simulink model "BESTROBITCS_in_output2"  (R2019b)
settings: Solver=FixedStepAuto  StartTime=0.0  StopTime=inf  RelTol=1e-3
libraries: vexarmcortexlib x32, vexcommonlib x6
settings Model: ExtModeTrigDuration=25  Creator=nicoa  LastModifiedBy=nicoa
settings OptimizationCC: EnhancedBackFolding=on  PassReuseOutputArgsAs=Individual arguments  ZeroExternalMemoryAtStartup=off  ZeroInternalMemoryAtStartup=off  MaxStackSize=64  OptimizeBlockOrder=speed  DifferentSizesBufferReuse=on  OptimizationCustomize=off  EfficientTunableParamExpr=on
settings DebuggingCC: ParameterTunabilityLossMsg=error
settings HardwareCC: ProdBitPerPointer=32  ProdBitPerSizeT=32  ProdBitPerPtrDiffT=32  ProdLargestAtomicInteger=Long  ProdLargestAtomicFloat=Double  ProdWordSize=32  ProdHWDeviceType=ARM Compatible->ARM Cortex
settings SFSimCC: MATLABDynamicMemAlloc=off
settings RTWCC: SystemTargetFile=ert.tlc  HardwareBoard=ARM Cortex-based VEX Microcontroller  TLCOptions="-aInlineSetEventsForThisBaseRateFcn=TLC_FALSE -aSuppressMultiTaskScheduler=TLC_FALSE  -aRateBasedStepFcn=0"  TemplateMakefile=ert_default_tmf  GenerateReport=on  Toolchain=GNU Tools for VEX ARM Cortex  IncludeHyperlinkInReport=on  LaunchReport=on  GenerateTraceInfo=on  GenerateTraceReport=on  GenerateTraceReportSl=on  GenerateTraceReportSf=on  GenerateTraceReportEml=on
settings CodeAppCC: ForceParamTrailComments=on  IgnoreCustomStorageClasses=off  OperatorAnnotations=on  SimulinkDataObjDesc=on  SFDataObjDesc=on  InsertBlockDesc=on

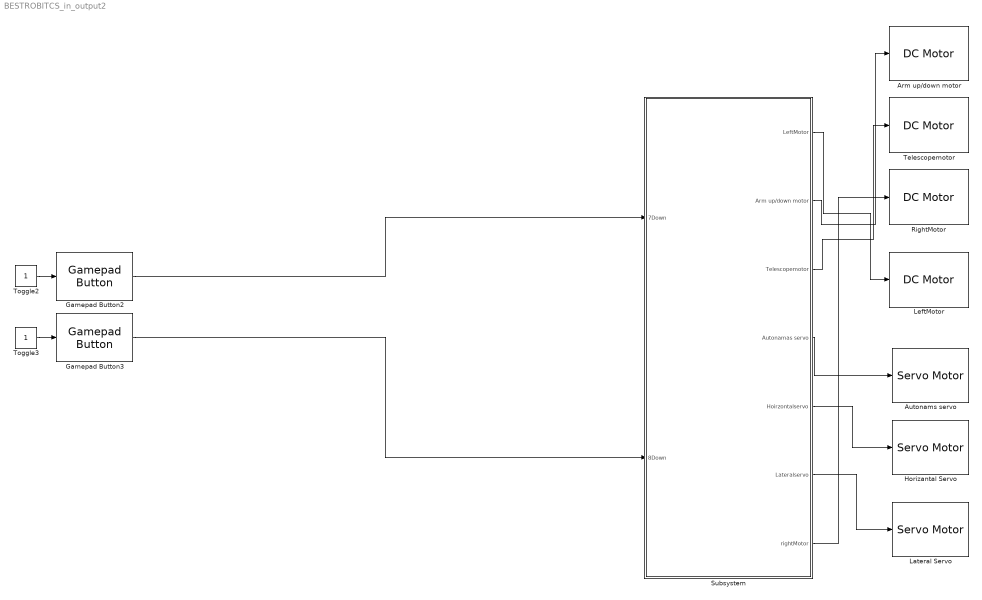
== system BESTROBITCS_in_output2 ==
  Arm up/down motor : vexarmcortexlib/Actuators/DC Motor  motor=7  scaleFactor=1/13.5  SimulationOut=on
      settings: SourceProductName=Simulink Coder Support Package for ARM Cortex-based VEX Microcontroller  SourceProductBaseCode=EC_VEX_MICRO
  Autonams servo : vexarmcortexlib/Actuators/Servo Motor  motor=5  scaleFactor=60/127  SimulationOut=on
      settings: SourceProductName=Simulink Coder Support Package for ARM Cortex-based VEX Microcontroller  SourceProductBaseCode=EC_VEX_MICRO
  Gamepad Button2 : vexarmcortexlib/Gamepad/Gamepad Button  joystick=1  chan=7  button56=Up  button78=Down  SimulationIn=on  SampleTime=0.02
      settings: SourceProductName=Simulink Coder Support Package for ARM Cortex-based VEX Microcontroller  SourceProductBaseCode=EC_VEX_MICRO
  Gamepad Button3 : vexarmcortexlib/Gamepad/Gamepad Button  joystick=1  chan=8  button56=Up  button78=Down  SimulationIn=on  SampleTime=0.02
      settings: SourceProductName=Simulink Coder Support Package for ARM Cortex-based VEX Microcontroller  SourceProductBaseCode=EC_VEX_MICRO
  Horizantal Servo : vexarmcortexlib/Actuators/Servo Motor  motor=2  scaleFactor=60/127  SimulationOut=on
      settings: SourceProductName=Simulink Coder Support Package for ARM Cortex-based VEX Microcontroller  SourceProductBaseCode=EC_VEX_MICRO
  Lateral Servo : vexarmcortexlib/Actuators/Servo Motor  motor=3  scaleFactor=60/127  SimulationOut=on
      settings: SourceProductName=Simulink Coder Support Package for ARM Cortex-based VEX Microcontroller  SourceProductBaseCode=EC_VEX_MICRO
  LeftMotor : vexarmcortexlib/Actuators/DC Motor  motor=9  scaleFactor=1/13.5  SimulationOut=off
      settings: SourceProductName=Simulink Coder Support Package for ARM Cortex-based VEX Microcontroller  SourceProductBaseCode=EC_VEX_MICRO
  RightMotor : vexarmcortexlib/Actuators/DC Motor  motor=4  scaleFactor=1/13.5  SimulationOut=on
      settings: SourceProductName=Simulink Coder Support Package for ARM Cortex-based VEX Microcontroller  SourceProductBaseCode=EC_VEX_MICRO
  Subsystem : Subsystem
  Telescopemotor : vexarmcortexlib/Actuators/DC Motor  motor=6  scaleFactor=1/13.5  SimulationOut=on
      settings: SourceProductName=Simulink Coder Support Package for ARM Cortex-based VEX Microcontroller  SourceProductBaseCode=EC_VEX_MICRO
  Toggle2 : Constant
      settings: OpenFcn=|
      | if strcmp('0',get_param(gcb, 'Value'))                        set_param(gcb, 'Value', '1');
      | else
      |             set_param(gcb, 'Value', '0');
      | end
  Toggle3 : Constant
      settings: OpenFcn=|
      | if strcmp('0',get_param(gcb, 'Value'))                        set_param(gcb, 'Value', '1');
      | else
      |             set_param(gcb, 'Value', '0');
      | end
  wires:
  Toggle2/1 -> Gamepad Button2/1
  Toggle3/1 -> Gamepad Button3/1
  Gamepad Button3/1 -> Subsystem/2(8Down)
  Gamepad Button2/1 -> Subsystem/1(7Down)
  Subsystem/1(LeftMotor) -> LeftMotor/1
  Subsystem/4(Autonamas servo) -> Autonams servo/1
  Subsystem/5(Hoirzontalservo) -> Horizantal Servo/1
  Subsystem/6(Lateralservo) -> Lateral Servo/1
  Subsystem/3("Telescopemotor ") -> Telescopemotor/1
  Subsystem/2(Arm up/down motor) -> Arm up/down motor/1
  Subsystem/7(rightMotor) -> RightMotor/1

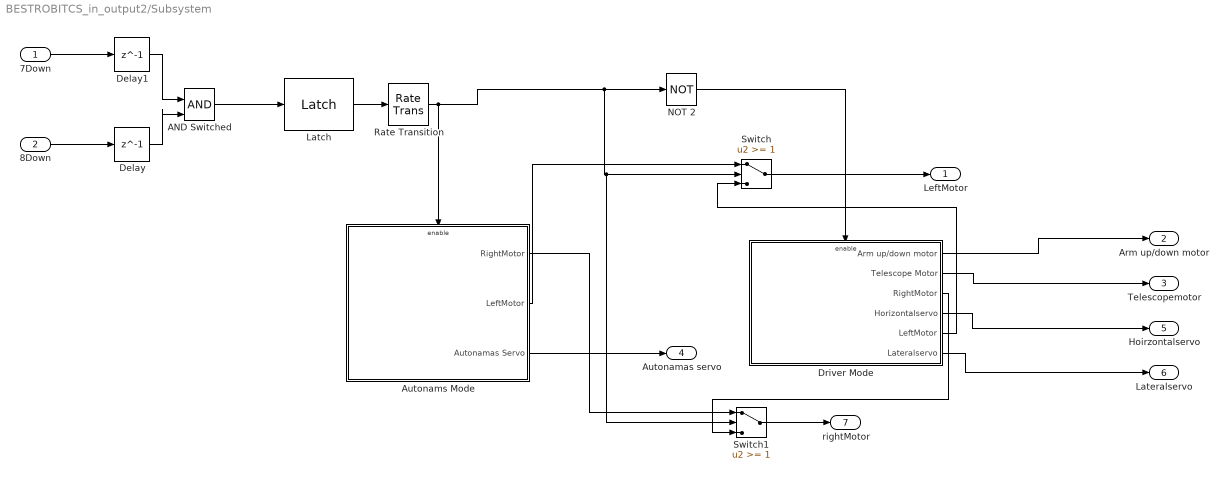
== system BESTROBITCS_in_output2/Subsystem ==
  7Down : Inport
  8Down : Inport  Port=2
  "AND Switched " : Logic  IconShape=distinctive  AllPortsSameDT=off  OutDataTypeStr=boolean
  Autonams Mode : Subsystem  TreatAsAtomicUnit=on
  Delay : Delay  DelayLength=1  InitialCondition=0  SampleTime=1
  Delay1 : Delay  DelayLength=1  InitialCondition=0  SampleTime=1
  "Driver Mode " : Subsystem  TreatAsAtomicUnit=on
  Latch : vexcommonlib/Latch  output0=off  BlockPlatform=vexarmcortex
      settings: SourceProductName=Simulink Coder Support Package for ARM Cortex-based VEX Microcontroller  SourceProductBaseCode=EC_VEX_MICRO
  NOT 2 : Logic  Operator=NOT  IconShape=distinctive  AllPortsSameDT=off  OutDataTypeStr=boolean
  Rate Transition : RateTransition
  Switch : Switch  Threshold=1
  Switch1 : Switch  Threshold=1
  LeftMotor : Outport
  Arm up/down motor : Outport  Port=2
  "Telescopemotor " : Outport  Port=3
  Autonamas servo : Outport  Port=4
  Hoirzontalservo : Outport  Port=5
  Lateralservo : Outport  Port=6
  rightMotor : Outport  Port=7
  wires:
  Delay/1 -> "AND Switched "/2
  Delay1/1 -> "AND Switched "/1
  Latch/1 -> Rate Transition/1
  8Down/1 -> Delay/1
  7Down/1 -> Delay1/1
  "AND Switched "/1 -> Latch/1
  Rate Transition/1 -> Switch1/2, Switch/2, NOT 2/1, Autonams Mode/Enable
  NOT 2/1 -> "Driver Mode "/Enable
  Autonams Mode/3(Autonamas Servo) -> Autonamas servo/1
  "Driver Mode "/4(Horizontalservo) -> Hoirzontalservo/1
  "Driver Mode "/6(Lateralservo) -> Lateralservo/1
  "Driver Mode "/2(Telescope Motor) -> "Telescopemotor "/1
  "Driver Mode "/1(Arm up/down motor) -> Arm up/down motor/1
  Autonams Mode/2(LeftMotor) -> Switch/1
  "Driver Mode "/5(LeftMotor) -> Switch/3
  Switch/1 -> LeftMotor/1
  Autonams Mode/1(RightMotor) -> Switch1/1
  "Driver Mode "/3(RightMotor) -> Switch1/3
  Switch1/1 -> rightMotor/1

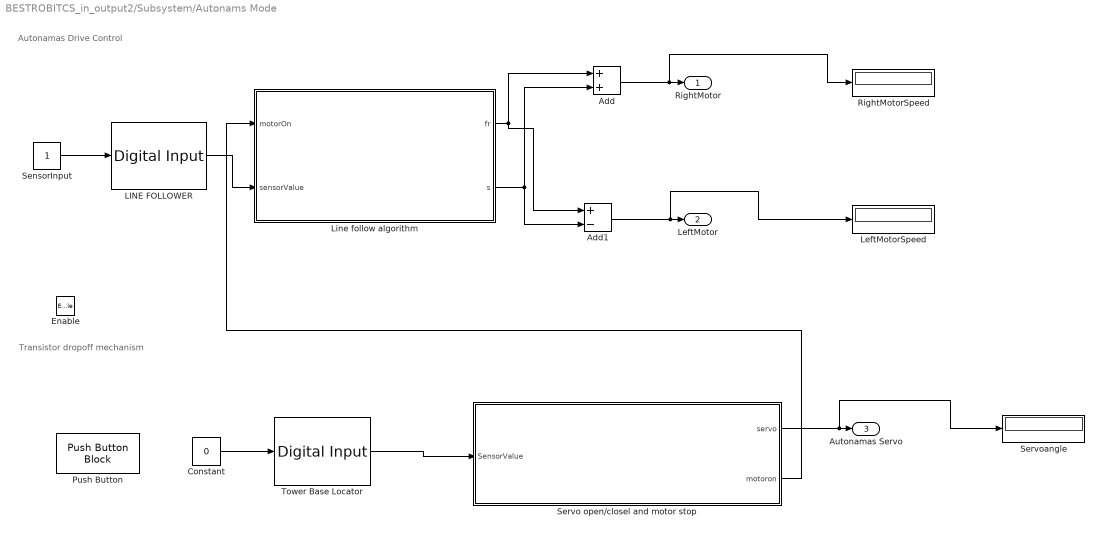
== system BESTROBITCS_in_output2/Subsystem/Autonams Mode ==
  note: Transistor dropoff mechanism
  note: Autonamas Drive Control
  Enable : EnablePort
  Add : Sum
  Add1 : Sum  Inputs=+-
  Constant : Constant  Value=0
  LINE FOLLOWER : vexarmcortexlib/Sensors/Digital Input  inChan=12  SimulationIn=on  SampleTime=0.2
      settings: SourceProductName=Simulink Coder Support Package for ARM Cortex-based VEX Microcontroller  SourceProductBaseCode=EC_VEX_MICRO
  LeftMotorSpeed : Display
  Line follow algorithm : Stateflow chart  TreatAsAtomicUnit=on
  Push Button : PushButtonBlock
  RightMotorSpeed : Display
  SensorInput : Constant
      settings: OpenFcn=|
      | if strcmp('0',get_param(gcb, 'Value'))                        set_param(gcb, 'Value', '1');
      | else
      |             set_param(gcb, 'Value', '0');
      | end
  Servo open/closel and motor stop : Stateflow chart  TreatAsAtomicUnit=on
  Servoangle : Display
  Tower Base Locator : vexarmcortexlib/Sensors/Digital Input  inChan=11  SimulationIn=on  SampleTime=0.2
      settings: SourceProductName=Simulink Coder Support Package for ARM Cortex-based VEX Microcontroller  SourceProductBaseCode=EC_VEX_MICRO
  RightMotor : Outport
  LeftMotor : Outport  Port=2
  Autonamas Servo : Outport  Port=3
  wires:
  Add/1 -> RightMotorSpeed/1, RightMotor/1
  Add1/1 -> LeftMotorSpeed/1, LeftMotor/1
  SensorInput/1 -> LINE FOLLOWER/1
  Line follow algorithm/2(s) -> Add1/2, Add/2
  Line follow algorithm/1(fr) -> Add1/1, Add/1
  Constant/1 -> Tower Base Locator/1
  Tower Base Locator/1 -> Servo open/closel and motor stop/1(SensorValue)
  Servo open/closel and motor stop/1(servo) -> Servoangle/1, Autonamas Servo/1
  LINE FOLLOWER/1 -> Line follow algorithm/2(sensorValue)
  Servo open/closel and motor stop/2(motoron) -> Line follow algorithm/1(motorOn)

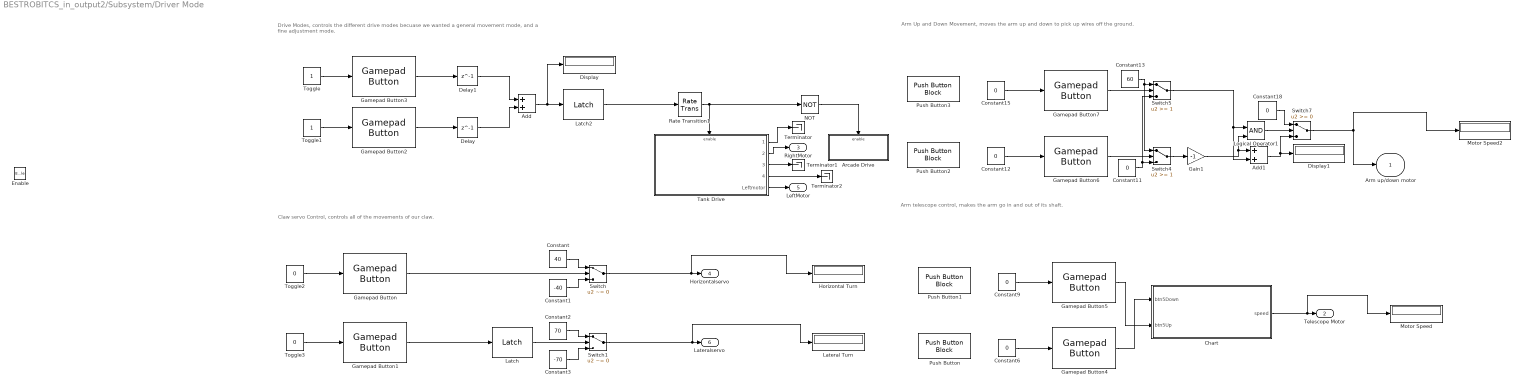
== system BESTROBITCS_in_output2/Subsystem/Driver Mode  ==
  note: Arm Up and Down Movement, moves the arm up and down to pick up wires off the ground.
  note: Arm telescope control, makes the arm go in and out of its shaft.
  note: Drive Modes, controls the different drive modes becuase we wanted a general movement mode, and a fine adjustment mode.
  note: Claw servo Control, controls all of the movements of our claw.
  Enable : EnablePort
  Add : Sum
  Add1 : Sum
  "Arcade Drive " : Subsystem  TreatAsAtomicUnit=on
  Chart : Stateflow chart  BlockKeywords=__PRM__SERIALIZED__DATA__:Stateflow Chart,Stateflow Diagram  TreatAsAtomicUnit=on
  Constant : Constant  Value=40
  Constant1 : Constant  Value=-40
  Constant{6,9,11..12,15,18} (6 alike) : Constant  Value=0
  Constant13 : Constant  Value=60
  Constant2 : Constant  Value=70
  Constant3 : Constant  Value=-70
  Delay : Delay  DelayLength=1  InitialCondition=0  SampleTime=1
  Delay1 : Delay  DelayLength=1  InitialCondition=0  SampleTime=1
  Display : Display
  Display1 : Display
  Gain1 : Gain  Gain=-1
  Gamepad Button : vexarmcortexlib/Gamepad/Gamepad Button  joystick=1  chan=8  button56=Up  button78=Up  SimulationIn=on  SampleTime=0.02
      settings: SourceProductName=Simulink Coder Support Package for ARM Cortex-based VEX Microcontroller  SourceProductBaseCode=EC_VEX_MICRO
  Gamepad Button1 : vexarmcortexlib/Gamepad/Gamepad Button  joystick=1  chan=7  button56=Up  button78=Up  SimulationIn=on  SampleTime=0.02
      settings: SourceProductName=Simulink Coder Support Package for ARM Cortex-based VEX Microcontroller  SourceProductBaseCode=EC_VEX_MICRO
  Gamepad Button2 : vexarmcortexlib/Gamepad/Gamepad Button  joystick=1  chan=8  button56=Up  button78=Left  SimulationIn=on  SampleTime=0.02
      settings: SourceProductName=Simulink Coder Support Package for ARM Cortex-based VEX Microcontroller  SourceProductBaseCode=EC_VEX_MICRO
  Gamepad Button3 : vexarmcortexlib/Gamepad/Gamepad Button  joystick=1  chan=7  button56=Up  button78=Left  SimulationIn=on  SampleTime=0.02
      settings: SourceProductName=Simulink Coder Support Package for ARM Cortex-based VEX Microcontroller  SourceProductBaseCode=EC_VEX_MICRO
  Gamepad Button4 : vexarmcortexlib/Gamepad/Gamepad Button  joystick=1  chan=5  button56=Down  button78=Down  SimulationIn=on  SampleTime=0.02
      settings: SourceProductName=Simulink Coder Support Package for ARM Cortex-based VEX Microcontroller  SourceProductBaseCode=EC_VEX_MICRO
  Gamepad Button5 : vexarmcortexlib/Gamepad/Gamepad Button  joystick=1  chan=5  button56=Up  button78=Down  SimulationIn=on  SampleTime=0.02
      settings: SourceProductName=Simulink Coder Support Package for ARM Cortex-based VEX Microcontroller  SourceProductBaseCode=EC_VEX_MICRO
  Gamepad Button6 : vexarmcortexlib/Gamepad/Gamepad Button  joystick=1  chan=6  button56=Down  button78=Down  SimulationIn=on  SampleTime=0.02
      settings: SourceProductName=Simulink Coder Support Package for ARM Cortex-based VEX Microcontroller  SourceProductBaseCode=EC_VEX_MICRO
  Gamepad Button7 : vexarmcortexlib/Gamepad/Gamepad Button  joystick=1  chan=6  button56=Up  button78=Down  SimulationIn=on  SampleTime=0.02
      settings: SourceProductName=Simulink Coder Support Package for ARM Cortex-based VEX Microcontroller  SourceProductBaseCode=EC_VEX_MICRO
  Horizontal Turn : Display
  Latch : vexcommonlib/Latch  output0=off  BlockPlatform=vexarmcortex
      settings: SourceProductName=Simulink Coder Support Package for ARM Cortex-based VEX Microcontroller  SourceProductBaseCode=EC_VEX_MICRO
  Latch2 : vexcommonlib/Latch  output0=off  BlockPlatform=vexarmcortex
      settings: SourceProductName=Simulink Coder Support Package for ARM Cortex-based VEX Microcontroller  SourceProductBaseCode=EC_VEX_MICRO
  Lateral Turn : Display
  Logical Operator1 : Logic  IconShape=distinctive  AllPortsSameDT=off  OutDataTypeStr=boolean
  Motor Speed : Display
  Motor Speed2 : Display
  NOT : Logic  Operator=NOT  IconShape=distinctive  AllPortsSameDT=off  OutDataTypeStr=boolean
  Push Button{,1..3} (4 alike) : PushButtonBlock
  Rate Transition1 : RateTransition
  Switch : Switch  Criteria=u2 ~= 0
  Switch1 : Switch  Criteria=u2 ~= 0
  Switch4 : Switch  Threshold=1
  Switch5 : Switch  Threshold=1
  Switch7 : Switch
  "Tank Drive " : Subsystem  TreatAsAtomicUnit=on
  Terminator : Terminator
  Terminator1 : Terminator
  Terminator2 : Terminator
  Toggle : Constant
      settings: OpenFcn=|
      | if strcmp('0',get_param(gcb, 'Value'))                        set_param(gcb, 'Value', '1');
      | else
      |             set_param(gcb, 'Value', '0');
      | end
  Toggle1 : Constant
      settings: OpenFcn=|
      | if strcmp('0',get_param(gcb, 'Value'))                        set_param(gcb, 'Value', '1');
      | else
      |             set_param(gcb, 'Value', '0');
      | end
  Toggle2 : Constant  Value=0
      settings: OpenFcn=|
      | if strcmp('0',get_param(gcb, 'Value'))                        set_param(gcb, 'Value', '1');
      | else
      |             set_param(gcb, 'Value', '0');
      | end
  Toggle3 : Constant  Value=0
      settings: OpenFcn=|
      | if strcmp('0',get_param(gcb, 'Value'))                        set_param(gcb, 'Value', '1');
      | else
      |             set_param(gcb, 'Value', '0');
      | end
  Arm up/down motor : Outport
  Telescope Motor : Outport  Port=2
  RightMotor : Outport  Port=3
  Horizontalservo : Outport  Port=4
  LeftMotor : Outport  Port=5
  Lateralservo : Outport  Port=6
  wires:
  Gamepad Button2/1 -> Delay/1
  Delay1/1 -> Add/1
  Gamepad Button3/1 -> Delay1/1
  Add/1 -> Display/1, Latch2/1
  Delay/1 -> Add/2
  Latch2/1 -> Rate Transition1/1
  NOT/1 -> "Arcade Drive "/Enable
  Switch/1 -> Horizontal Turn/1, Horizontalservo/1
  Switch1/1 -> Lateral Turn/1, Lateralservo/1
  Constant1/1 -> Switch/3
  Constant/1 -> Switch/1
  Gamepad Button/1 -> Switch/2
  Gamepad Button1/1 -> Latch/1
  Constant2/1 -> Switch1/1
  Constant3/1 -> Switch1/3
  Latch/1 -> Switch1/2
  Toggle1/1 -> Gamepad Button2/1
  Toggle/1 -> Gamepad Button3/1
  Rate Transition1/1 -> NOT/1, "Tank Drive "/Enable
  Toggle2/1 -> Gamepad Button/1
  Toggle3/1 -> Gamepad Button1/1
  Chart/1(speed) -> Motor Speed/1, Telescope Motor/1
  Switch4/1 -> Gain1/1
  Gamepad Button7/1 -> Switch5/2
  Gamepad Button6/1 -> Switch4/2
  Switch7/1 -> Motor Speed2/1, Arm up/down motor/1
  Constant11/1 -> Switch5/3, Switch4/3
  Constant13/1 -> Switch4/1, Switch5/1
  Switch5/1 -> Add1/2, Logical Operator1/1
  Gain1/1 -> Logical Operator1/2, Add1/1
  Logical Operator1/1 -> Switch7/2
  Constant18/1 -> Switch7/1
  Add1/1 -> Display1/1, Switch7/3
  Gamepad Button4/1 -> Chart/1(btn5Down)
  Gamepad Button5/1 -> Chart/2(btn5Up)
  Constant6/1 -> Gamepad Button4/1
  Constant9/1 -> Gamepad Button5/1
  Constant15/1 -> Gamepad Button7/1
  Constant12/1 -> Gamepad Button6/1
  "Tank Drive "/5("Leftmotor ") -> LeftMotor/1
  "Tank Drive "/2 -> RightMotor/1
  "Tank Drive "/1 -> Terminator/1
  "Tank Drive "/3 -> Terminator1/1
  "Tank Drive "/4 -> Terminator2/1

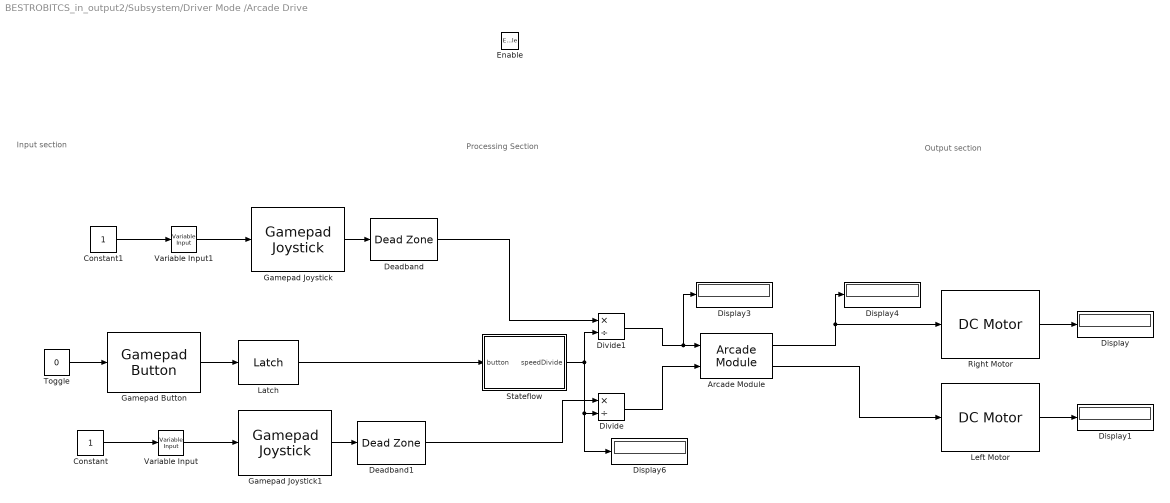
== system BESTROBITCS_in_output2/Subsystem/Driver Mode /Arcade Drive  ==
  note: Output section
  note: Processing Section
  note: Input section
  Enable : EnablePort
  Arcade Module : vexcommonlib/Arcade Module  BlockPlatform=vexarmcortex
      settings: SourceProductName=Simulink Coder Support Package for ARM Cortex-based VEX Microcontroller  SourceProductBaseCode=EC_VEX_MICRO
  Constant : Constant
  Constant1 : Constant
  Deadband : DeadZone  LowerValue=-5  UpperValue=5  SaturateOnIntegerOverflow=on
  Deadband1 : DeadZone  LowerValue=-5  UpperValue=5  SaturateOnIntegerOverflow=on
  Display{,1,3..4,6} (5 alike) : Display
  Divide : Product  Inputs=*/
  Divide1 : Product  Inputs=*/
  Gamepad Button : vexarmcortexlib/Gamepad/Gamepad Button  joystick=1  chan=8  button56=Up  button78=Down  SimulationIn=on  SampleTime=0.02
      settings: SourceProductName=Simulink Coder Support Package for ARM Cortex-based VEX Microcontroller  SourceProductBaseCode=EC_VEX_MICRO
  Gamepad Joystick : vexarmcortexlib/Gamepad/Gamepad Joystick  joystick=1  chan=2  SimulationIn=on  SampleTime=0.02
      settings: SourceProductName=Simulink Coder Support Package for ARM Cortex-based VEX Microcontroller  SourceProductBaseCode=EC_VEX_MICRO
  Gamepad Joystick1 : vexarmcortexlib/Gamepad/Gamepad Joystick  joystick=1  chan=1  SimulationIn=on  SampleTime=0.02
      settings: SourceProductName=Simulink Coder Support Package for ARM Cortex-based VEX Microcontroller  SourceProductBaseCode=EC_VEX_MICRO
  Latch : vexcommonlib/Latch  output0=off  BlockPlatform=vexarmcortex
      settings: SourceProductName=Simulink Coder Support Package for ARM Cortex-based VEX Microcontroller  SourceProductBaseCode=EC_VEX_MICRO
  Left Motor : vexarmcortexlib/Actuators/DC Motor  motor=9  scaleFactor=1/13.5  SimulationOut=on
      settings: SourceProductName=Simulink Coder Support Package for ARM Cortex-based VEX Microcontroller  SourceProductBaseCode=EC_VEX_MICRO
  Right Motor : vexarmcortexlib/Actuators/DC Motor  motor=8  scaleFactor=1/13.5  SimulationOut=on
      settings: SourceProductName=Simulink Coder Support Package for ARM Cortex-based VEX Microcontroller  SourceProductBaseCode=EC_VEX_MICRO
  Stateflow : Stateflow chart  TreatAsAtomicUnit=on
  Toggle : Constant  Value=0
      settings: OpenFcn=|
      | if strcmp('0',get_param(gcb, 'Value'))                        set_param(gcb, 'Value', '1');
      | else
      |             set_param(gcb, 'Value', '0');
      | end
  Variable Input : vexarmcortexlib/Utilities/Variable Input  low=-127  gain=16.9723  high=127
      settings: SourceProductName=Simulink Coder Support Package for ARM Cortex-based VEX Microcontroller  SourceProductBaseCode=EC_VEX_MICRO
  Variable Input1 : vexarmcortexlib/Utilities/Variable Input  low=-127  gain=-5.2672  high=127
      settings: SourceProductName=Simulink Coder Support Package for ARM Cortex-based VEX Microcontroller  SourceProductBaseCode=EC_VEX_MICRO
  wires:
  Arcade Module/2 -> Left Motor/1
  Gamepad Joystick1/1 -> Deadband1/1
  Arcade Module/1 -> Display4/1, Right Motor/1
  Gamepad Joystick/1 -> Deadband/1
  Gamepad Button/1 -> Latch/1
  Stateflow/1(speedDivide) -> Display6/1, Divide/2, Divide1/2
  Deadband/1 -> Divide1/1
  Deadband1/1 -> Divide/1
  Divide/1 -> Arcade Module/2
  Divide1/1 -> Display3/1, Arcade Module/1
  Right Motor/1 -> Display/1
  Left Motor/1 -> Display1/1
  Latch/1 -> Stateflow/1(button)
  Variable Input/1 -> Gamepad Joystick1/1
  Constant/1 -> Variable Input/1
  Constant1/1 -> Variable Input1/1
  Variable Input1/1 -> Gamepad Joystick/1
  Toggle/1 -> Gamepad Button/1

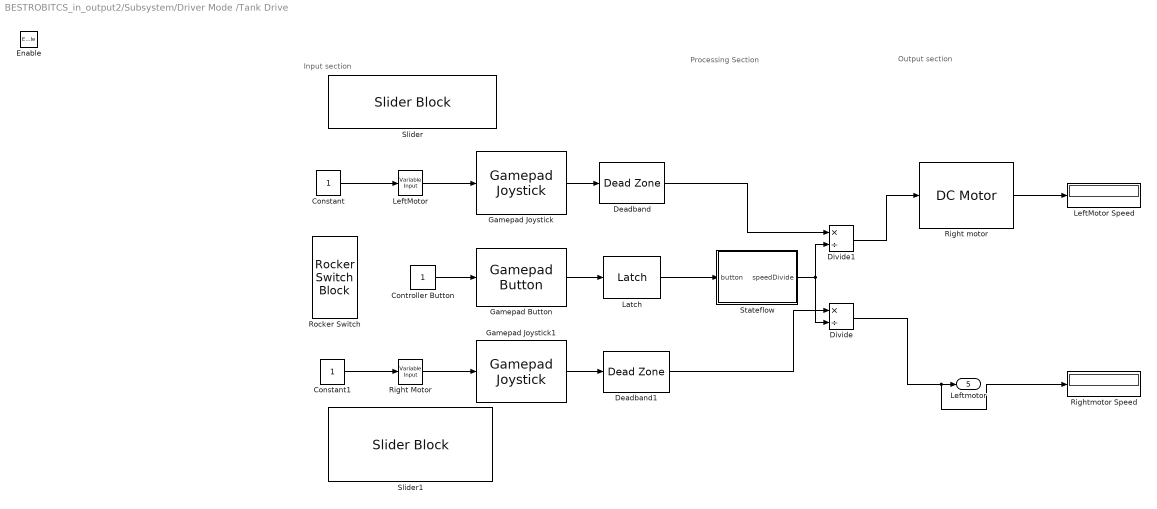
== system BESTROBITCS_in_output2/Subsystem/Driver Mode /Tank Drive  ==
  note: Output section
  note: Processing Section
  note: Input section
  Enable : EnablePort
  Constant : Constant
  Constant1 : Constant
  Controller Button : Constant
  Deadband : DeadZone  LowerValue=-5  UpperValue=5  SaturateOnIntegerOverflow=on
  Deadband1 : DeadZone  LowerValue=-5  UpperValue=5  SaturateOnIntegerOverflow=on
  Divide : Product  Inputs=*/
  Divide1 : Product  Inputs=*/
  Gamepad Button : vexarmcortexlib/Gamepad/Gamepad Button  joystick=1  chan=8  button56=Down  button78=Down  SimulationIn=on  SampleTime=0.02
      settings: SourceProductName=Simulink Coder Support Package for ARM Cortex-based VEX Microcontroller  SourceProductBaseCode=EC_VEX_MICRO
  Gamepad Joystick : vexarmcortexlib/Gamepad/Gamepad Joystick  joystick=1  chan=3  SimulationIn=on  SampleTime=0.02
      settings: SourceProductName=Simulink Coder Support Package for ARM Cortex-based VEX Microcontroller  SourceProductBaseCode=EC_VEX_MICRO
  Gamepad Joystick1 : vexarmcortexlib/Gamepad/Gamepad Joystick  joystick=1  chan=2  SimulationIn=on  SampleTime=0.02
      settings: SourceProductName=Simulink Coder Support Package for ARM Cortex-based VEX Microcontroller  SourceProductBaseCode=EC_VEX_MICRO
  Latch : vexcommonlib/Latch  output0=off  BlockPlatform=vexarmcortex
      settings: SourceProductName=Simulink Coder Support Package for ARM Cortex-based VEX Microcontroller  SourceProductBaseCode=EC_VEX_MICRO
  LeftMotor : vexarmcortexlib/Utilities/Variable Input  low=-127  gain=6.704272598870062  high=127
      settings: SourceProductName=Simulink Coder Support Package for ARM Cortex-based VEX Microcontroller  SourceProductBaseCode=EC_VEX_MICRO
  LeftMotor Speed : Display
  Right Motor : vexarmcortexlib/Utilities/Variable Input  low=-127  gain=-77.96239406779661  high=127
      settings: SourceProductName=Simulink Coder Support Package for ARM Cortex-based VEX Microcontroller  SourceProductBaseCode=EC_VEX_MICRO
  "Right motor " : vexarmcortexlib/Actuators/DC Motor  motor=8  scaleFactor=1/13.5  SimulationOut=on
      settings: SourceProductName=Simulink Coder Support Package for ARM Cortex-based VEX Microcontroller  SourceProductBaseCode=EC_VEX_MICRO
  Rightmotor Speed : Display
  Rocker Switch : RockerSwitchBlock
      settings: Values={{'Off', 'On'}, [0 1]}
  Slider : SliderBlock  ScaleMin=-127  ScaleMax=127
  Slider1 : SliderBlock  ScaleMin=-127  ScaleMax=127
  Stateflow : Stateflow chart  TreatAsAtomicUnit=on
  "Leftmotor " : Outport  Port=5
  wires:
  Gamepad Joystick/1 -> Deadband/1
  Gamepad Joystick1/1 -> Deadband1/1
  Gamepad Button/1 -> Latch/1
  Latch/1 -> Stateflow/1(button)
  Stateflow/1(speedDivide) -> Divide1/2, Divide/2
  Deadband/1 -> Divide1/1
  Divide1/1 -> "Right motor "/1
  Deadband1/1 -> Divide/1
  Constant/1 -> LeftMotor/1
  LeftMotor/1 -> Gamepad Joystick/1
  Constant1/1 -> Right Motor/1
  Right Motor/1 -> Gamepad Joystick1/1
  Controller Button/1 -> Gamepad Button/1
  "Right motor "/1 -> LeftMotor Speed/1
  Divide/1 -> Rightmotor Speed/1, "Leftmotor "/1

== stateflow chart BESTROBITCS_in_output2/Subsystem/Autonams Mode/Line follow algorithm ==
  state GO_RIGHT
    entry:
    fr = 50;
    s = -50;
  state GO_LEFT
    entry:
    fr = 50;
    s = 50;
  state STOPPED
    entry:
    fr = 0;
    s = 0;
  (default) -> GO_LEFT
  GO_LEFT -> GO_RIGHT [order 2] : [sensorValue == 1]
  GO_RIGHT -> GO_LEFT [order 2] : [sensorValue == 0]
  GO_LEFT -> STOPPED [order 1] : [motorOn == 0]
  GO_RIGHT -> STOPPED [order 1] : [motorOn == 0]
  data: fr output; s output; motorOn input; sensorValue input

== stateflow chart BESTROBITCS_in_output2/Subsystem/Driver Mode /Arcade Drive /Stateflow ==
  state Full_Speed
    entry:
    speedDivide = 1
  state Slow_Speed
    entry:
    speedDivide = 4
  (default) -> Full_Speed
  Full_Speed -> Slow_Speed : [button == 1]
  Slow_Speed -> Full_Speed : [button == 0]
  data: speedDivide output; button input

== stateflow chart BESTROBITCS_in_output2/Subsystem/Driver Mode /Tank Drive /Stateflow ==
  state Full_Speed
    entry:
    speedDivide = 1
  state Slow_Speed
    entry:
    speedDivide = 4
  (default) -> Full_Speed
  Full_Speed -> Slow_Speed : [button]
  Slow_Speed -> Full_Speed : [button == 0]
  data: speedDivide output; button input

== stateflow chart BESTROBITCS_in_output2/Subsystem/Autonams Mode/Servo open//closel and motor stop ==
  state move
    entry:
    servo = 0;
    motoron = 1;
  state Stop
    entry:
    servo = 67;
    motoron = 0;
  state off
    entry:
    servo = 0;
    motoron = 0;
  (default) -> move
  move -> Stop : [SensorValue == 1]
  Stop -> off : [after(300,sec)]
  data: SensorValue input; servo output; motoron output

== stateflow chart BESTROBITCS_in_output2/Subsystem/Driver Mode /Chart ==
  state ARMDOWN
    entry:
    speed = -40;
  state STOPPED
    entry:
    speed = 0;
  state ARMUP
    entry:
    speed = 40;
  (default) -> STOPPED
  STOPPED -> ARMUP [order 1] : [btn5Down ==-0 && btn5Up == 1 ]
  STOPPED -> ARMDOWN [order 2] : [btn5Down == 1 && btn5Up == 0]
  ARMDOWN -> STOPPED [order 1] : [btn5Down == 0]
  ARMUP -> STOPPED [order 1] : [btn5Up == 0]
  ARMDOWN -> STOPPED [order 2] : [btn5Up == 1]
  ARMUP -> STOPPED [order 2] : [btn5Down == 1]
  data: btn5Down input; btn5Up input; speed output
